simulink model "sim_01_b_RightSide_dynamic"  (R2022a)
settings: Solver=VariableStepAuto  StartTime=0.0  StopTime=50  RelTol=1e-3
settings Model: Creator=Eshmith  LastModifiedBy=Eshmith

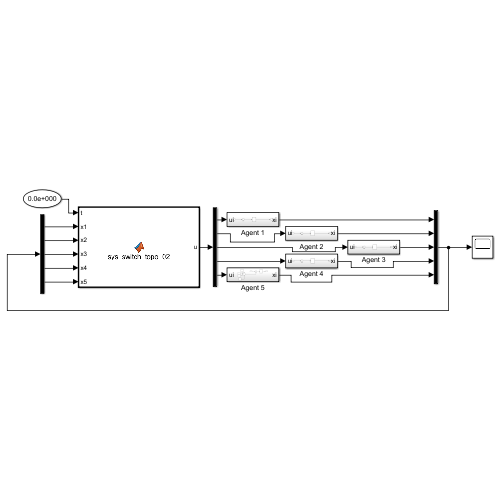
[thumbnail: Simulink's stored preview of the top-level diagram]
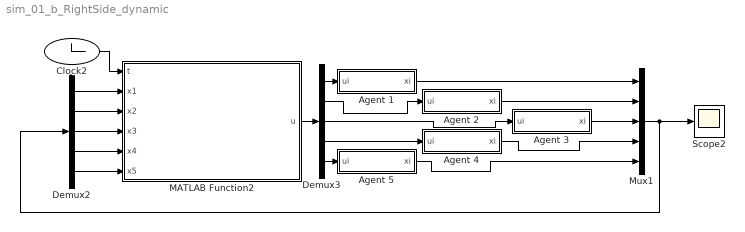
== system sim_01_b_RightSide_dynamic ==
  Agent 1 : Subsystem
  Agent 2 : Subsystem
  Agent 3 : Subsystem
  Agent 4 : Subsystem
  Agent 5 : Subsystem
  Clock2 : Clock
  Demux2 : Demux  Outputs=5
  Demux3 : Demux  Outputs=5
  MATLAB Function2 : MATLAB Function  TreatAsAtomicUnit=on
  Mux1 : Mux  Inputs=5
  Scope2 : Scope
  wires:
  Demux3/3 -> Agent 3/1(ui)
  MATLAB Function2/1(u) -> Demux3/1
  Demux3/2 -> Agent 2/1(ui)
  Agent 3/1(xi) -> Mux1/3
  Demux3/1 -> Agent 1/1(ui)
  Demux2/4 -> MATLAB Function2/5(x4)
  Demux3/5 -> Agent 5/1(ui)
  Mux1/1 -> Demux2/1, Scope2/1
  Agent 5/1(xi) -> Mux1/5
  Demux2/5 -> MATLAB Function2/6(x5)
  Demux2/2 -> MATLAB Function2/3(x2)
  Demux2/3 -> MATLAB Function2/4(x3)
  Demux2/1 -> MATLAB Function2/2(x1)
  Agent 1/1(xi) -> Mux1/1
  Demux3/4 -> Agent 4/1(ui)
  Agent 4/1(xi) -> Mux1/4
  Agent 2/1(xi) -> Mux1/2
  Clock2/1 -> MATLAB Function2/1(t)

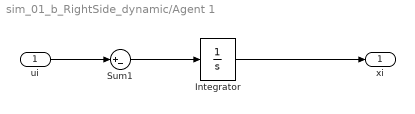
== system sim_01_b_RightSide_dynamic/Agent 1 ==
  ui : Inport
  Integrator : Integrator  InitialCondition=4
  Sum1 : Sum  Inputs=|+-
  xi : Outport
  wires:
  Sum1/1 -> Integrator/1
  ui/1 -> Sum1/1
  Integrator/1 -> xi/1

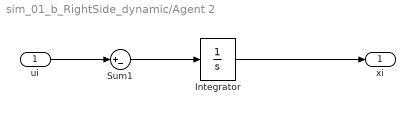
== system sim_01_b_RightSide_dynamic/Agent 2 ==
  ui : Inport
  Integrator : Integrator  InitialCondition=1
  Sum1 : Sum  Inputs=|+-
  xi : Outport
  wires:
  Sum1/1 -> Integrator/1
  ui/1 -> Sum1/1
  Integrator/1 -> xi/1

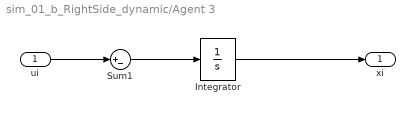
== system sim_01_b_RightSide_dynamic/Agent 3 ==
  ui : Inport
  Integrator : Integrator  InitialCondition=2
  Sum1 : Sum  Inputs=|+-
  xi : Outport
  wires:
  Sum1/1 -> Integrator/1
  ui/1 -> Sum1/1
  Integrator/1 -> xi/1

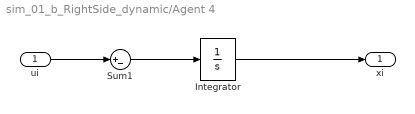
== system sim_01_b_RightSide_dynamic/Agent 4 ==
  ui : Inport
  Integrator : Integrator  InitialCondition=3
  Sum1 : Sum  Inputs=|+-
  xi : Outport
  wires:
  Sum1/1 -> Integrator/1
  ui/1 -> Sum1/1
  Integrator/1 -> xi/1

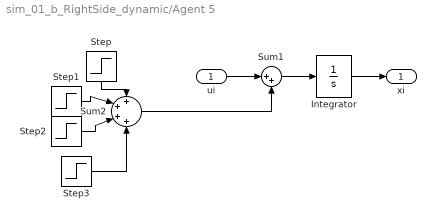
== system sim_01_b_RightSide_dynamic/Agent 5 ==
  ui : Inport
  Integrator : Integrator  InitialCondition=10
  Step : Step  Time=20  SampleTime=0
  Step1 : Step  Time=25  After=-0.5  SampleTime=0
  Step2 : Step  Time=30  After=-1  SampleTime=0
  Step3 : Step  Time=35  After=0.5  SampleTime=0
  Sum1 : Sum  Inputs=|++
  Sum2 : Sum  Inputs=++++
  xi : Outport
  wires:
  Sum1/1 -> Integrator/1
  ui/1 -> Sum1/1
  Integrator/1 -> xi/1
  Step1/1 -> Sum2/2
  Step2/1 -> Sum2/3
  Step/1 -> Sum2/1
  Sum2/1 -> Sum1/2
  Step3/1 -> Sum2/4

== matlab function sim_01_b_RightSide_dynamic/MATLAB Function2 ==
  data: t input; x1 input; u output; x2 input; x3 input; x4 input; x5 input
function u = sys_switch_topo_02(t, x1, x2, x3, x4, x5)

if rem(floor(t/2),2) == 0
    L = [2  0 -1  0 -1;
         0  0  0  0  0;
         0  0  0  0  0;
         0  0 -1 +1  0;
         0  0  0  0  0;
        ];

else
    L = [2 -1  0  0 -1;
         0  0  0  0  0;
         0  0  0  0  0;
         0 -1  0 +1  0;
         0  0  0  0  0;
        ];
end
    
states = [x1, x2, x3, x4 x5]';

u = -L*states;

end
